simulink model "calories"  (R2022b)
settings: Solver=VariableStepAuto  StartTime=0.0  StopTime=3000.0  RelTol=1e-3
libraries: cstblocks x1
settings Model: Creator=integzz  LastModifiedBy=integzz

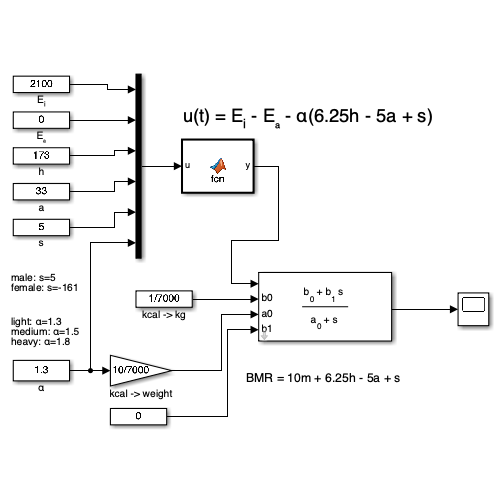
[thumbnail: Simulink's stored preview of the top-level diagram]
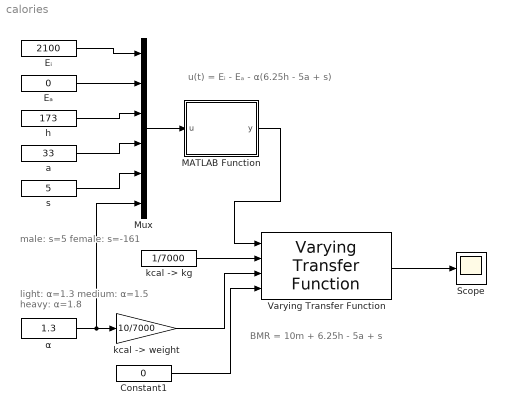
== system calories ==
  note: u(t) = Eᵢ - Eₐ - α(6.25h - 5a + s)
  note: male: s=5
      | female: s=-161
  note: light: α=1.3
      | medium: α=1.5
      | heavy: α=1.8
  note: BMR = 10m + 6.25h - 5a + s
  Constant1 : Constant  Value=0
  Eᵢ : Constant  Value=2100
  Eₐ : Constant  Value=0
  MATLAB Function : MATLAB Function  TreatAsAtomicUnit=on
  Mux : Mux  Inputs=6
  Scope : Scope
  Varying Transfer Function : cstblocks/Linear Parameter Varying/Varying Transfer Function  N=1
      link override Integrator1: InitialCondition=71.5
  a : Constant  Value=33
  h : Constant  Value=173
  "kcal -> kg" : Constant  Value=1/7000
  "kcal -> weight" : Gain  Gain=10/7000
  s : Constant  Value=5
  α : Constant  Value=1.3
  wires:
  "kcal -> kg"/1 -> Varying Transfer Function/2
  "kcal -> weight"/1 -> Varying Transfer Function/3
  Constant1/1 -> Varying Transfer Function/4
  Eᵢ/1 -> Mux/1
  Eₐ/1 -> Mux/2
  h/1 -> Mux/3
  a/1 -> Mux/4
  s/1 -> Mux/5
  Mux/1 -> MATLAB Function/1(u)
  α/1 -> Mux/6, "kcal -> weight"/1
  MATLAB Function/1(y) -> Varying Transfer Function/1
  Varying Transfer Function/1 -> Scope/1

== matlab function calories/MATLAB Function ==
  data: u input; y output
function y = fcn(u)

y = u(1)-u(2)-u(6)*(6.25*u(3)-5*u(4)+u(5));
